simulink model "Subsystem"  (R2020b)
settings: Solver=VariableStepAuto  StartTime=0.0  StopTime=10.0  RelTol=1e-3
undefined symbols (not defined in the file): Ki, Kp, Ts
settings Model: Creator=pawankumarf  LastModifiedBy=admin
settings DataIOCC: ExternalInput=[t, stin]  LoadExternalInput=on  SaveFormat=Array  SaveOutput=off  SaveTime=off  ReturnWorkspaceOutputs=off

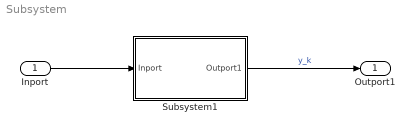
== system Subsystem ==
  Inport : Inport  OutDataTypeStr=double  PortDimensions=1  SampleTime=0
  Subsystem1 : Subsystem  TreatAsAtomicUnit=on
  Outport1 : Outport  OutDataTypeStr=double  PortDimensions=1  SampleTime=0
  wires:
  Inport/1 -> Subsystem1/1(Inport)
  Subsystem1/1(Outport1) -> Outport1/1  "y_k"

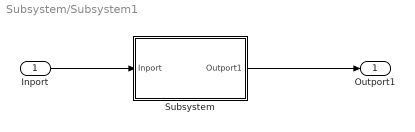
== system Subsystem/Subsystem1 ==
  Inport : Inport
  Subsystem : Subsystem
  Outport1 : Outport
  wires:
  Inport/1 -> Subsystem/1(Inport)
  Subsystem/1(Outport1) -> Outport1/1

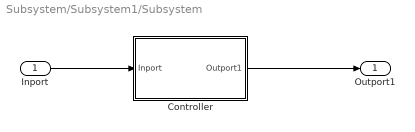
== system Subsystem/Subsystem1/Subsystem ==
  Inport : Inport
  Controller : Subsystem  TreatAsAtomicUnit=on
  Outport1 : Outport
  wires:
  Inport/1 -> Controller/1(Inport)
  Controller/1(Outport1) -> Outport1/1

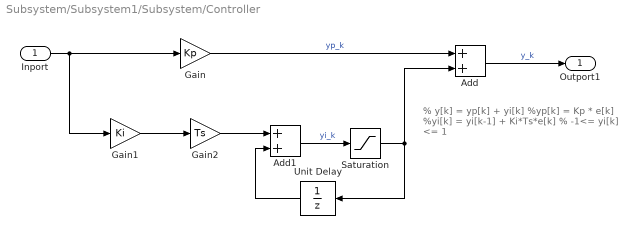
== system Subsystem/Subsystem1/Subsystem/Controller ==
  note: % y[k] = yp[k] + yi[k]
      | %yp[k] = Kp * e[k]
      | %yi[k] = yi[k-1] + Ki*Ts*e[k]
      | % -1<= yi[k] <= 1
  Inport : Inport
  Add : Sum
  Add1 : Sum
  Gain : Gain  Gain=Kp
  Gain1 : Gain  Gain=Ki
  Gain2 : Gain  Gain=Ts
  Saturation : Saturate  UpperLimit=1  LowerLimit=-1
  Unit Delay : UnitDelay  SampleTime=-1  HasFrameUpgradeWarning=on
  Outport1 : Outport
  wires:
  Add1/1 -> Saturation/1  "yi_k"
  Saturation/1 -> Unit Delay/1, Add/2
  Unit Delay/1 -> Add1/2
  Gain1/1 -> Gain2/1
  Inport/1 -> Gain/1, Gain1/1
  Add/1 -> Outport1/1  "y_k"
  Gain2/1 -> Add1/1
  Gain/1 -> Add/1  "yp_k"
